simulink model "Buck"  (R2024b)
settings: Solver=FixedStepAuto  StartTime=0.0  StopTime=1.5e-3  FixedStep=100e-9  RelTol=1e-3
InitFcn:
  | Vin = 100;
  | 
  | R = 13.3;
  | L = 420e-6;
  | C = 8e-6;
  | 
  | overL = 1/L;
  | overR = 1/R;
  | overC = 1/C;
  | 
  | fs = 20e3;
  | D = 50;
  | 
  | h = double(1e-6);
settings Model: Creator=User  LastModifiedBy=User

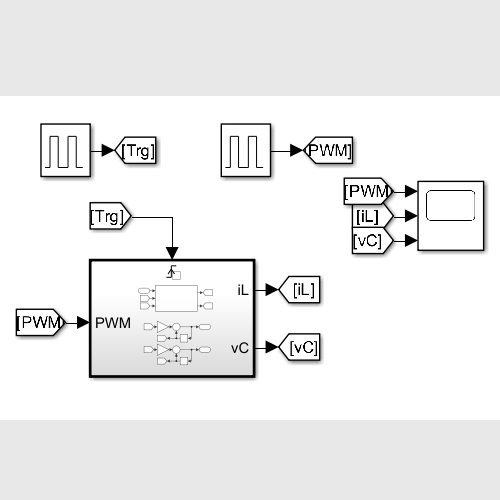
[thumbnail: Simulink's stored preview of the top-level diagram]
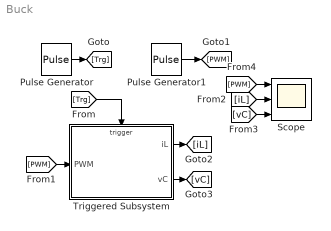
== system Buck ==
  Pulse Generator : DiscretePulseGenerator  PulseType=Time based  Period=1e-6  PulseWidth=10
  Pulse Generator1 : DiscretePulseGenerator  PulseType=Time based  Period=1/fs  PulseWidth=D
  Scope : Scope  NumInputPorts=3
  Triggered Subsystem : Subsystem  TreatAsAtomicUnit=on
  wires:
  [Trg] -> Triggered Subsystem/Trigger
  [PWM] -> Triggered Subsystem/1(PWM)
  Triggered Subsystem/1(iL) -> [iL]
  Triggered Subsystem/2(vC) -> [vC]
  [iL] -> Scope/2
  [vC] -> Scope/3
  [PWM] -> Scope/1
  Pulse Generator1/1 -> [PWM]
  Pulse Generator/1 -> [Trg]

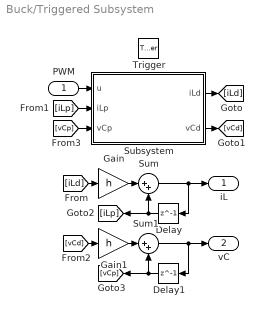
== system Buck/Triggered Subsystem ==
  PWM : Inport
  Trigger : TriggerPort  VariantControl=(inherit)
  Delay : Delay  DelayLength=1
  Delay1 : Delay  DelayLength=1
  Gain : Gain  Gain=h
  Gain1 : Gain  Gain=h
  Subsystem : Subsystem
  Sum : Sum  Inputs=|++  OutDataTypeStr=single
  Sum1 : Sum  Inputs=|++  OutDataTypeStr=single
  iL : Outport
  vC : Outport  Port=2
  wires:
  Delay/1 -> [iLp], Sum/2
  Sum/1 -> Delay/1, iL/1
  Sum1/1 -> vC/1, Delay1/1
  PWM/1 -> Subsystem/1(u)
  Subsystem/1(iLd) -> [iLd]
  Subsystem/2(vCd) -> [vCd]
  Gain/1 -> Sum/1
  [iLd] -> Gain/1
  [iLp] -> Subsystem/2(iLp)
  Gain1/1 -> Sum1/1
  [vCd] -> Gain1/1
  [vCp] -> Subsystem/3(vCp)
  Delay1/1 -> Sum1/2, [vCp]

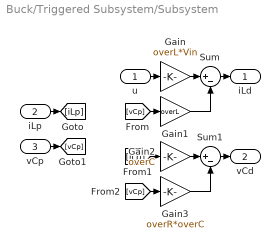
== system Buck/Triggered Subsystem/Subsystem ==
  u : Inport
  iLp : Inport  Port=2
  vCp : Inport  Port=3
  Gain : Gain  Gain=overL*Vin
  Gain1 : Gain  Gain=overL
  Gain2 : Gain  Gain=overC
  Gain3 : Gain  Gain=overR*overC
  Sum : Sum  Inputs=|+-  OutDataTypeStr=single
  Sum1 : Sum  Inputs=|+-  OutDataTypeStr=single
  iLd : Outport
  vCd : Outport  Port=2
  wires:
  iLp/1 -> [iLp]
  vCp/1 -> [vCp]
  Gain/1 -> Sum/1
  u/1 -> Gain/1
  Sum/1 -> iLd/1
  [vCp] -> Gain1/1
  Gain1/1 -> Sum/2
  Sum1/1 -> vCd/1
  [iLp] -> Gain2/1
  Gain2/1 -> Sum1/1
  [vCp] -> Gain3/1
  Gain3/1 -> Sum1/2
